simulink model "RoomRadiator_Compare"  (R2013b)
settings: Solver=ode23t  StartTime=0.0  StopTime=24*3600  RelTol=1e-3
undefined symbols (not defined in the file): density, heat_capacity
libraries: carnot x60, simulink x4, simulink_extras x2
settings Model: Creator=drhf  LastModifiedBy=drhf
settings OptimizationCC: ExpressionDepthLimit=2147483647
settings DebuggingCC: StateNameClashWarn=warning
settings GRTTargetCC: CombineOutputUpdateFcns=off  GRTInterface=on

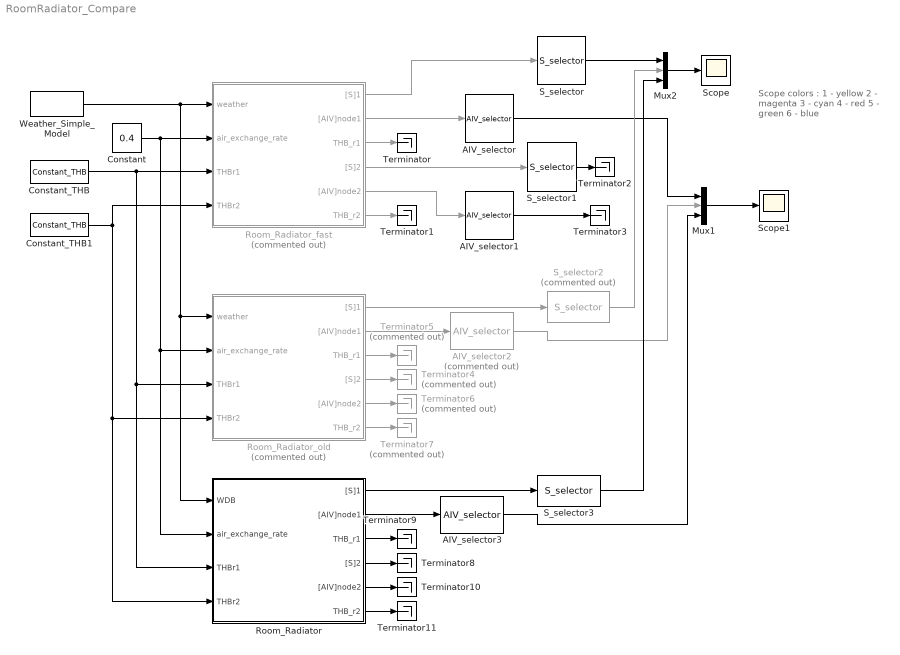
== system RoomRadiator_Compare ==
  note: Scope colors :
      | 1 - yellow
      | 2 - magenta
      | 3 - cyan
      | 4 - red
      | 5 - green
      | 6 - blue
  AIV_selector : carnot/Outputs/AIV_selector  e1=on  e2=on  e3=on  e4=off  e5=off  e6=off  e7=off  e8=off  e9=off
  AIV_selector1 : carnot/Outputs/AIV_selector  e1=on  e2=on  e3=on  e4=off  e5=off  e6=off  e7=off  e8=off  e9=off
  AIV_selector2 : carnot/Outputs/AIV_selector  Commented=on  e1=on  e2=on  e3=on  e4=off  e5=off  e6=off  e7=off  e8=off  e9=off
  AIV_selector3 : carnot/Outputs/AIV_selector  e1=on  e2=on  e3=on  e4=off  e5=off  e6=off  e7=off  e8=off  e9=off
  Constant : Constant  Value=0.4
  Constant_THB : carnot/Source/Simple/Constant_THB  t=30  mdot=600/3600  p=1e5  mID=No Pressure Drop  fluid=Water  mix=0  dia=0.02  hgt=0
  Constant_THB1 : carnot/Source/Simple/Constant_THB  t=40  mdot=600/3600  p=1e5  mID=No Pressure Drop  fluid=Water  mix=0  dia=0.02  hgt=0
  Mux1 : Mux  Inputs=3
  Mux2 : Mux  Inputs=3
  Room_Radiator : Subsystem  AncestorBlock=carnot/Load/Houses/Room_Radiator  mask(room){t0=20, temp_neighbour=20}
      mask prompts: t0 "start temperature of rooms in °C"; temp_neighbour "temperature of rooms above and below in °C"
      mask help:
      | The block models of a heat transfer characteristic of two neighbour rooms.
      | Use "look under mask" to set up the models parameters (initial conditions,
      | floors and wall characteristics...)
      mask init:
      | AIV_neighbour = [0 temp_neighbour temp_neighbour 0 0 0 0 0 0];
      | zonefloordist2grnd = 0;
      mask Help: web(fullfile(path_carnot('help'),'Room_Radiator.html'),'-helpbrowser')
      mask Display: plot(0,0,100,100,[30,30,60,60,30],[20,50,50,20,20],[47,47,56,56,47],[40,30,30,40,40],[42,42,34,34],[20,40,40,20],[62,45,28],[48,70,48])
  Room_Radiator_fast : Subsystem  Commented=on  AncestorBlock=carnot/Load/Houses/Room_Radiator  mask(room){t0=20, temp_neighbour=20}
      mask prompts: t0 "start temperature of rooms in °C"; temp_neighbour "temperature of rooms above and below in °C"
      mask help:
      | The block models of a heat transfer characteristic of two neighbour rooms.
      | Use "look under mask" to set up the models parameters (initial conditions,
      | floors and wall characteristics...)
      mask init:
      | AIV_neighbour = [0 temp_neighbour temp_neighbour 0 0 0 0 0 0];
      | zonefloordist2grnd = 0;
      mask Help: eval('man(''room_radiator'')')
      mask Display: plot(0,0,100,100,[30,30,60,60,30],[20,50,50,20,20],[47,47,56,56,47],[40,30,30,40,40],[42,42,34,34],[20,40,40,20],[62,45,28],[48,70,48])
  Room_Radiator_old : Subsystem  Commented=on  AncestorBlock=carnot/Load/Houses/Room_Radiator  mask(room){t0=20, temp_neighbour=20}
      mask prompts: t0 "start temperature of rooms in °C"; temp_neighbour "temperature of rooms above and below in °C"
      mask help:
      | The block models of a heat transfer characteristic of two neighbour rooms.
      | Use "look under mask" to set up the models parameters (initial conditions,
      | floors and wall characteristics...)
      mask init:
      | AIV_neighbour = [0 temp_neighbour temp_neighbour 0 0 0 0 0 0];
      | zonefloordist2grnd = 0;
      mask Help: eval('man(''room_radiator'')')
      mask Display: plot(0,0,100,100,[30,30,60,60,30],[20,50,50,20,20],[47,47,56,56,47],[40,30,30,40,40],[42,42,34,34],[20,40,40,20],[62,45,28],[48,70,48])
  S_selector : carnot/Outputs/S_selector  e1=off  e2=off  e3=off  e4=off  e5=off  e6=off  e7=on  e8=on  e9=off  e10=off  e11=off  e12=off  e13=off
  S_selector1 : carnot/Outputs/S_selector  e1=off  e2=off  e3=off  e4=off  e5=off  e6=off  e7=on  e8=on  e9=off  e10=off  e11=off  e12=off  e13=off
  S_selector2 : carnot/Outputs/S_selector  Commented=on  e1=off  e2=off  e3=off  e4=off  e5=off  e6=off  e7=on  e8=on  e9=off  e10=off  e11=off  e12=off  e13=off
  S_selector3 : carnot/Outputs/S_selector  e1=off  e2=off  e3=off  e4=off  e5=off  e6=off  e7=on  e8=on  e9=off  e10=off  e11=off  e12=off  e13=off
  Scope : Scope
      settings: YMin=0  YMax=12
  Scope1 : Scope
  Terminator{,1..3,8..11} (8 alike) : Terminator
  Terminator{4..7} (4 alike) : Terminator  Commented=on
  Weather_Simple_Model : carnot/Weather/Weather_Simple_Model  lat=60  Ibn=900  Idg=100  tamb=5  deltaTsky=-6  rh=50  precip="10e-3/24/3600           % 10 mm in 24 h"  cloud=0.125  p=1013e2  vw=1  wdir=270
  wires:
  Weather_Simple_Model/1 -> Room_Radiator_old/1(weather), Room_Radiator/1(WDB), Room_Radiator_fast/1(weather)
  Constant/1 -> Room_Radiator_old/2(air_exchange_rate), Room_Radiator/2(air_exchange_rate), Room_Radiator_fast/2(air_exchange_rate)
  Constant_THB/1 -> Room_Radiator_old/3(THBr1), Room_Radiator/3(THBr1), Room_Radiator_fast/3(THBr1)
  Constant_THB1/1 -> Room_Radiator_old/4(THBr2), Room_Radiator/4(THBr2), Room_Radiator_fast/4(THBr2)
  Room_Radiator_fast/1("[S]1") -> S_selector/1
  Room_Radiator_fast/2("[AIV]node1") -> AIV_selector/1
  Room_Radiator_fast/5("[AIV]node2") -> AIV_selector1/1
  Room_Radiator_fast/4("[S]2") -> S_selector1/1
  Room_Radiator_fast/3(THB_r1) -> Terminator/1
  Room_Radiator_fast/6(THB_r2) -> Terminator1/1
  Mux1/1 -> Scope1/1
  AIV_selector/1 -> Mux1/1
  S_selector1/1 -> Terminator2/1
  S_selector/1 -> Mux2/1
  Mux2/1 -> Scope/1
  Room_Radiator_old/1("[S]1") -> S_selector2/1
  S_selector2/1 -> Mux2/2
  AIV_selector1/1 -> Terminator3/1
  Room_Radiator_old/4("[S]2") -> Terminator4/1
  Room_Radiator_old/3(THB_r1) -> Terminator5/1
  Room_Radiator_old/5("[AIV]node2") -> Terminator6/1
  Room_Radiator_old/6(THB_r2) -> Terminator7/1
  Room_Radiator_old/2("[AIV]node1") -> AIV_selector2/1
  AIV_selector2/1 -> Mux1/2
  Room_Radiator/4("[S]2") -> Terminator8/1
  Room_Radiator/3(THB_r1) -> Terminator9/1
  Room_Radiator/5("[AIV]node2") -> Terminator10/1
  Room_Radiator/6(THB_r2) -> Terminator11/1
  Room_Radiator/2("[AIV]node1") -> AIV_selector3/1
  Room_Radiator/1("[S]1") -> S_selector3/1
  S_selector3/1 -> Mux2/3
  AIV_selector3/1 -> Mux1/3

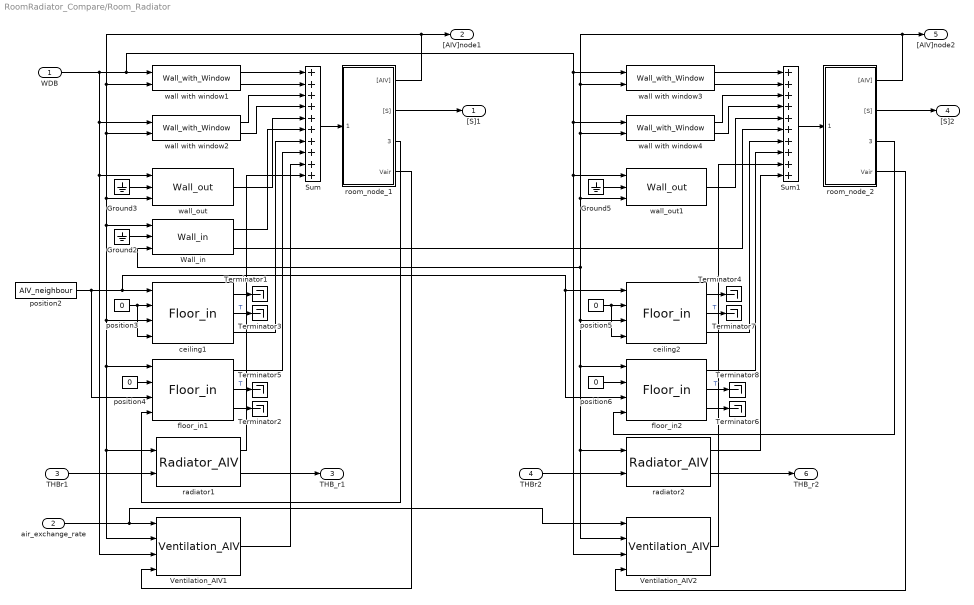
== system RoomRadiator_Compare/Room_Radiator ==
  WDB : Inport
  air_exchange_rate : Inport  Port=2
  THBr1 : Inport  Port=3
  THBr2 : Inport  Port=4
  Ground2 : Ground
  Ground3 : Ground
  Ground5 : Ground
  Sum : Sum  Inputs=10  SaturateOnIntegerOverflow=on  InputSameDT=on  OutDataTypeStr=Inherit: Same as first input
  Sum1 : Sum  Inputs=10  SaturateOnIntegerOverflow=on  InputSameDT=on  OutDataTypeStr=Inherit: Same as first input
  Terminator{1..8} (8 alike) : Terminator
  Ventilation_AIV1 : carnot/Source/Ventilation/Ventilation_AIV  co2=400
  Ventilation_AIV2 : carnot/Source/Ventilation/Ventilation_AIV  co2=400
  Wall_in : carnot/Load/Houses/wall_floor/Wall_in  wallsize=[2.5 5]  d=[0.015 0.38 0.02]  cond=[1.4 0.79 0.7]  cwall=[0.28 0.28 0.28]*3600  rho=[2000 1800 1400]  emission_in=0.96  dactive=-1  t0=20  tau=1000*3600
  ceiling1 : carnot/Load/Houses/wall_floor/Floor_in  wallsize=[5 5]  t0=20  d=[0.015 0.38 0.02]  cond=[1.4 0.79 0.7]  cwall=[0.28 0.28 0.28]*3600  rho=[2000 1800 1400]  misc=[.65 .65]  dactive=-1  tau=1000*3600
  ceiling2 : carnot/Load/Houses/wall_floor/Floor_in  wallsize=[5 5]  t0=20  d=[0.015 0.38 0.02]  cond=[1.4 0.79 0.7]  cwall=[0.28 0.28 0.28]*3600  rho=[2000 1800 1400]  misc=[.65 .65]  dactive=-1  tau=1000*3600
  floor_in1 : carnot/Load/Houses/wall_floor/Floor_in  wallsize=[5 5]  t0=20  d=[0.015 0.38 0.02]  cond=[1.4 0.79 0.7]  cwall=[0.28 0.28 0.28]*3600  rho=[2000 1800 1400]  misc=[.65 .65]  dactive=-1  tau=1000*3600
  floor_in2 : carnot/Load/Houses/wall_floor/Floor_in  wallsize=[5 5]  t0=20  d=[0.015 0.38 0.02]  cond=[1.4 0.79 0.7]  cwall=[0.28 0.28 0.28]*3600  rho=[2000 1800 1400]  misc=[.65 .65]  dactive=-1  tau=1000*3600
  position2 : Constant  Value=AIV_neighbour
  position{3..6} (4 alike) : Constant  Value=0
  radiator1 : carnot/Source/Heat_Exchanger/Radiator_AIV  pnom=500  dtnom=40  expo=1.3  mcap=5*4182  ra=0.47  tini=20  lin=0  qua=1000
  radiator2 : carnot/Source/Heat_Exchanger/Radiator_AIV  pnom=500  dtnom=40  expo=1.3  mcap=5*4182  ra=0.47  tini=20  lin=0  qua=1000
  room_node_1 : Subsystem  AncestorBlock=carnot/Load/Houses/room_node/Room_Node  mask(NODE){zoneairvolume=5*5*2.5, zoneheight=2.5, zonestartTEMP=20, zonestartWATER=55, timeconst=100, heatperfect=natural, lookuptime=[0 24]*3600, lookupvalue=[20 20], AirPressure=101300}
      mask prompts: zoneairvolume "SIZE: netto air volume >0, m^3"; zoneheight "SIZE: height of zone (floor - ceiling) >0, m"; zonestartTEMP "START TEMPERATURE: convective and radiative node, °C"; zonestartWATER "START AIR HUMIDITY: relative air humidity [0,100], %"; timeconst "timeconstant of radiative and convective node in s"; heatperfect "air temperature"; lookuptime "time vector for ideal profile [s]"; lookupvalue "values for ideal profile [degree centigrade]"; AirPressure "Air pressure for material properties in Pa"
      mask help:
      | This block delivers the energy consumption, temperature and air quality of a zone.
      | It is assumed that this node represents the center of a zone all connected sink and source blocks communicate with. Sink and source blocks are walls, windows, persons, heater etc..
      | Properties of air are calculated once at initialization (with node start temperature, humidity and air pressure).
      | [S] : input vector from sink blocks and source blocks
      | [AIV] : output vector with node temperature and air quality data.
      mask init:
      | CO2norm = 400*1e-6;
      | zoneairvolume = max(0.01, zoneairvolume);
      | zoneheight = max(0.01, zoneheight);
      | zonestartWATER = min(100, max(0, zonestartWATER));
      | zonestartWATER = rel_hum2x(zonestartTEMP, 10^5, zonestartWATER)*1.18*zoneairvolume; % kg H2O in zone volume (at 20°C)
      | zonestartCO2 = CO2norm*1.529*zoneairvolume; % kg CO2 in zone volume
      | zonestartAIR = 10^5*zoneairvolume/(287*(zonestartTEMP+273)); % kg AIR in zone volume
      mask Help: web(fullfile(path_carnot('help'),'Room_Node.html'),'-helpbrowser')
      mask TypeOptions heatperfect: natural | ideal profile (for heating demand)
  room_node_2 : Subsystem  AncestorBlock=carnot/Load/Houses/room_node/Room_Node  mask(NODE){zoneairvolume=5*5*2.5, zoneheight=2.5, zonestartTEMP=20, zonestartWATER=55, timeconst=100, heatperfect=natural, lookuptime=[0 24]*3600, lookupvalue=[20 20], AirPressure=101300}
      mask prompts: zoneairvolume "SIZE: netto air volume >0, m^3"; zoneheight "SIZE: height of zone (floor - ceiling) >0, m"; zonestartTEMP "START TEMPERATURE: convective and radiative node, °C"; zonestartWATER "START AIR HUMIDITY: relative air humidity [0,100], %"; timeconst "timeconstant of radiative and convective node in s"; heatperfect "air temperature"; lookuptime "time vector for ideal profile [s]"; lookupvalue "values for ideal profile [degree centigrade]"; AirPressure "Air pressure for material properties in Pa"
      mask help:
      | This block delivers the energy consumption, temperature and air quality of a zone.
      | It is assumed that this node represents the center of a zone all connected sink and source blocks communicate with. Sink and source blocks are walls, windows, persons, heater etc..
      | Properties of air are calculated once at initialization (with node start temperature, humidity and air pressure).
      | [S] : input vector from sink blocks and source blocks
      | [AIV] : output vector with node temperature and air quality data.
      mask init: same as RoomRadiator_Compare/Room_Radiator/room_node_1
      mask Help: web(fullfile(path_carnot('help'),'Room_Node.html'),'-helpbrowser')
      mask TypeOptions heatperfect: natural | ideal profile (for heating demand)
  wall with window1 : carnot/Load/Houses/wall_floor/Wall_with_Window  wallsize=[2.5 5]  windowsize=[1 2]  frame=0.1  pos=90  t0=20  tau=1000*3600  g=0.7
  wall with window2 : carnot/Load/Houses/wall_floor/Wall_with_Window  wallsize=[2.5 5]  windowsize=[1 2]  frame=0.1  pos=0  t0=20  tau=1000*3600  g=0.7
  wall with window3 : carnot/Load/Houses/wall_floor/Wall_with_Window  wallsize=[2.5 5]  windowsize=[1 2]  frame=0.1  pos=-90  t0=20  tau=1000*3600  g=0.7
  wall with window4 : carnot/Load/Houses/wall_floor/Wall_with_Window  wallsize=[2.5 5]  windowsize=[1 2]  frame=0.1  pos=0  t0=20  tau=1000*3600  g=0.7
  wall_out : carnot/Load/Houses/wall_floor/Wall_out  wallsize=[2.5 5]  pos=180  t0=20  d=[0.1 0.38]  cond=[0.04 0.79]  cwall=[0.28 0.28]*3600  rho=[900 1800]  reflectground=0.2  abs_emiss=[0.65 0.97 0.96]  tau=1000*3600  dactive=-1
  wall_out1 : carnot/Load/Houses/wall_floor/Wall_out  wallsize=[2.5 5]  pos=180  t0=20  d=[0.1 0.38]  cond=[0.04 0.79]  cwall=[0.28 0.28]*3600  rho=[900 1800]  reflectground=0.2  abs_emiss=[0.65 0.97 0.96]  tau=1000*3600  dactive=-1
  "[S]1" : Outport
  "[AIV]node1" : Outport  Port=2
  THB_r1 : Outport  Port=3
  "[S]2" : Outport  Port=4
  "[AIV]node2" : Outport  Port=5
  THB_r2 : Outport  Port=6
  wires:
  Sum1/1 -> room_node_2/1(sum([S]))
  Sum/1 -> room_node_1/1(sum([S]))
  radiator2/1 -> Sum1/10
  radiator1/1 -> Sum/10
  position6/1 -> floor_in2/2
  position4/1 -> floor_in1/2
  floor_in1/2 -> Terminator5/1  "T"
  floor_in2/2 -> Terminator8/1  "T"
  room_node_2/1("[AIV]") -> "[AIV]node2"/1, wall with window3/2, wall with window4/2, Wall_in/3, ceiling2/3, Ventilation_AIV2/2, radiator2/1, floor_in2/1, wall_out1/3
  room_node_1/1("[AIV]") -> "[AIV]node1"/1, wall_out/3, Wall_in/1, Ventilation_AIV1/2, radiator1/1, floor_in1/1, ceiling1/3, wall with window2/2, wall with window1/2
  air_exchange_rate/1 -> Ventilation_AIV2/1, Ventilation_AIV1/1
  Wall_in/2 -> Sum1/6
  Ground5/1 -> wall_out1/2
  room_node_2/3(Qdot_sol) -> floor_in2/4
  room_node_2/4(Vair) -> Ventilation_AIV2/4
  radiator2/2 -> THB_r2/1
  THBr2/1 -> radiator2/2
  Ventilation_AIV2/1 -> Sum1/9
  ceiling2/3 -> Sum1/7
  floor_in2/1 -> Sum1/8
  position5/1 -> ceiling2/2, ceiling2/4
  floor_in2/3 -> Terminator6/1
  ceiling2/2 -> Terminator7/1  "T"
  ceiling2/1 -> Terminator4/1
  room_node_2/2("[S]") -> "[S]2"/1
  wall with window4/2 -> Sum1/4
  wall_out1/1 -> Sum1/5
  wall with window4/1 -> Sum1/3
  wall with window3/2 -> Sum1/2
  wall with window3/1 -> Sum1/1
  position2/1 -> floor_in2/3, ceiling2/1, ceiling1/1, floor_in1/3
  Ground3/1 -> wall_out/2
  Ground2/1 -> Wall_in/2
  room_node_1/3(Qdot_sol) -> floor_in1/4
  room_node_1/4(Vair) -> Ventilation_AIV1/4
  radiator1/2 -> THB_r1/1
  THBr1/1 -> radiator1/2
  Ventilation_AIV1/1 -> Sum/9
  ceiling1/3 -> Sum/7
  floor_in1/1 -> Sum/8
  position3/1 -> ceiling1/4, ceiling1/2
  floor_in1/3 -> Terminator2/1
  ceiling1/2 -> Terminator3/1  "T"
  ceiling1/1 -> Terminator1/1
  room_node_1/2("[S]") -> "[S]1"/1
  wall with window2/2 -> Sum/4
  wall_out/1 -> Sum/5
  wall with window2/1 -> Sum/3
  wall with window1/2 -> Sum/2
  wall with window1/1 -> Sum/1
  WDB/1 -> wall with window3/1, wall with window4/1, Ventilation_AIV2/3, wall_out1/1, wall with window1/1, Ventilation_AIV1/3, wall_out/1, wall with window2/1
  Wall_in/1 -> Sum/6

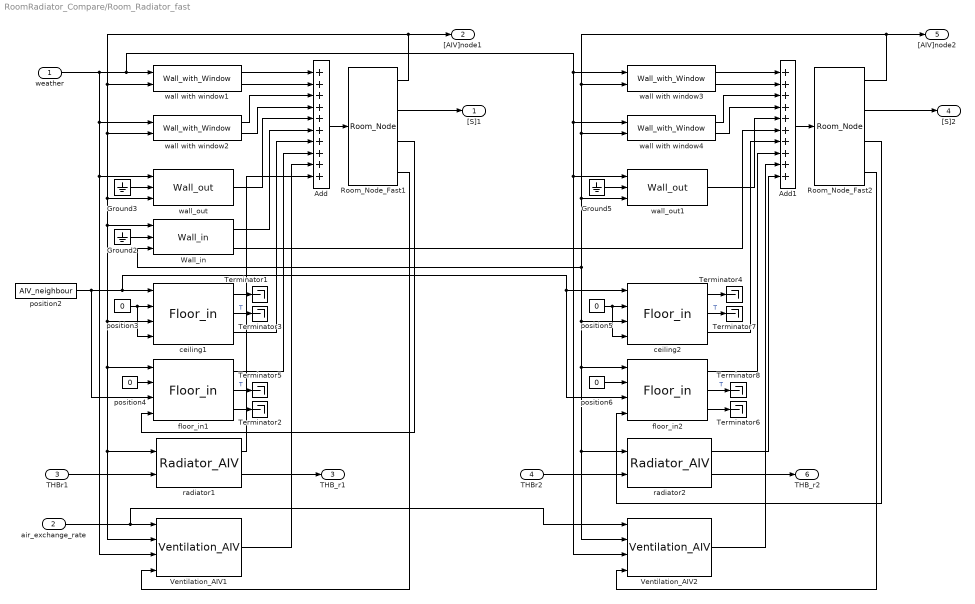
== system RoomRadiator_Compare/Room_Radiator_fast ==
  weather : Inport
  air_exchange_rate : Inport  Port=2
  THBr1 : Inport  Port=3
  THBr2 : Inport  Port=4
  Add : Sum  Inputs=10
  Add1 : Sum  Inputs=10
  Ground2 : Ground
  Ground3 : Ground
  Ground5 : Ground
  Room_Node_Fast1 : carnot/Load/Houses/room_node/Room_Node  zoneairvolume=5*5*2.5  zoneheight=2.5  zonestartTEMP=20  zonestartWATER=55  timeconst=100  heatperfect=natural  lookuptime=[0 7 7 20 20 24]*3600  lookupvalue=[18 18 20 20 18 18]  AirPressure=101300
  Room_Node_Fast2 : carnot/Load/Houses/room_node/Room_Node  zoneairvolume=5*5*2.5  zoneheight=2.5  zonestartTEMP=20  zonestartWATER=55  timeconst=100  heatperfect=natural  lookuptime=[0 7 7 20 20 24]*3600  lookupvalue=[18 18 20 20 18 18]  AirPressure=101300
  Terminator{1..8} (8 alike) : Terminator
  Ventilation_AIV1 : carnot/Source/Ventilation/Ventilation_AIV  co2=400
  Ventilation_AIV2 : carnot/Source/Ventilation/Ventilation_AIV  co2=400
  Wall_in : carnot/Load/Houses/wall_floor/Wall_in  wallsize=[2.5 5]  d=[0.015 0.38 0.02]  cond=[1.4 0.79 0.7]  cwall=[0.28 0.28 0.28]*3600  rho=[2000 1800 1400]  emission_in=0.96  dactive=-1  t0=20  tau=1000*3600
  ceiling1 : carnot/Load/Houses/wall_floor/Floor_in  wallsize=[5 5]  t0=20  d=[0.015 0.38 0.02]  cond=[1.4 0.79 0.7]  cwall=[0.28 0.28 0.28]*3600  rho=[2000 1800 1400]  misc=[.65 .65]  dactive=-1  tau=1000*3600
  ceiling2 : carnot/Load/Houses/wall_floor/Floor_in  wallsize=[5 5]  t0=20  d=[0.015 0.38 0.02]  cond=[1.4 0.79 0.7]  cwall=[0.28 0.28 0.28]*3600  rho=[2000 1800 1400]  misc=[.65 .65]  dactive=-1  tau=1000*3600
  floor_in1 : carnot/Load/Houses/wall_floor/Floor_in  wallsize=[5 5]  t0=20  d=[0.015 0.38 0.02]  cond=[1.4 0.79 0.7]  cwall=[0.28 0.28 0.28]*3600  rho=[2000 1800 1400]  misc=[.65 .65]  dactive=-1  tau=1000*3600
  floor_in2 : carnot/Load/Houses/wall_floor/Floor_in  wallsize=[5 5]  t0=20  d=[0.015 0.38 0.02]  cond=[1.4 0.79 0.7]  cwall=[0.28 0.28 0.28]*3600  rho=[2000 1800 1400]  misc=[.65 .65]  dactive=-1  tau=1000*3600
  position2 : Constant  Value=AIV_neighbour
  position{3..6} (4 alike) : Constant  Value=0
  radiator1 : carnot/Source/Heat_Exchanger/Radiator_AIV  pnom=500  dtnom=40  expo=1.3  mcap=5*4182  ra=0.47  tini=20  lin=0  qua=1000
  radiator2 : carnot/Source/Heat_Exchanger/Radiator_AIV  pnom=500  dtnom=40  expo=1.3  mcap=5*4182  ra=0.47  tini=20  lin=0  qua=1000
  wall with window1 : carnot/Load/Houses/wall_floor/Wall_with_Window  wallsize=[2.5 5]  windowsize=[1 2]  frame=0.1  pos=90  t0=20  tau=1000*3600  g=0.7
  wall with window2 : carnot/Load/Houses/wall_floor/Wall_with_Window  wallsize=[2.5 5]  windowsize=[1 2]  frame=0.1  pos=0  t0=20  tau=1000*3600  g=0.7
  wall with window3 : carnot/Load/Houses/wall_floor/Wall_with_Window  wallsize=[2.5 5]  windowsize=[1 2]  frame=0.1  pos=-90  t0=20  tau=1000*3600  g=0.7
  wall with window4 : carnot/Load/Houses/wall_floor/Wall_with_Window  wallsize=[2.5 5]  windowsize=[1 2]  frame=0.1  pos=0  t0=20  tau=1000*3600  g=0.7
  wall_out : carnot/Load/Houses/wall_floor/Wall_out  wallsize=[2.5 5]  pos=180  t0=20  d=[0.1 0.38]  cond=[0.04 0.79]  cwall=[0.28 0.28]*3600  rho=[900 1800]  reflectground=0.2  abs_emiss=[0.65 0.97 0.96]  tau=1000*3600  dactive=-1
  wall_out1 : carnot/Load/Houses/wall_floor/Wall_out  wallsize=[2.5 5]  pos=180  t0=20  d=[0.1 0.38]  cond=[0.04 0.79]  cwall=[0.28 0.28]*3600  rho=[900 1800]  reflectground=0.2  abs_emiss=[0.65 0.97 0.96]  tau=1000*3600  dactive=-1
  "[S]1" : Outport
  "[AIV]node1" : Outport  Port=2
  THB_r1 : Outport  Port=3
  "[S]2" : Outport  Port=4
  "[AIV]node2" : Outport  Port=5
  THB_r2 : Outport  Port=6
  wires:
  radiator2/1 -> Add1/10
  radiator1/1 -> Add/10
  position6/1 -> floor_in2/2
  position4/1 -> floor_in1/2
  floor_in1/2 -> Terminator5/1  "T"
  floor_in2/2 -> Terminator8/1  "T"
  Room_Node_Fast2/1 -> wall with window3/2, wall with window4/2, Wall_in/3, ceiling2/3, Ventilation_AIV2/2, radiator2/1, floor_in2/1, wall_out1/3, "[AIV]node2"/1
  Room_Node_Fast1/1 -> wall_out/3, Wall_in/1, Ventilation_AIV1/2, radiator1/1, floor_in1/1, ceiling1/3, wall with window2/2, wall with window1/2, "[AIV]node1"/1
  air_exchange_rate/1 -> Ventilation_AIV2/1, Ventilation_AIV1/1
  Wall_in/2 -> Add1/6
  Ground5/1 -> wall_out1/2
  Room_Node_Fast2/3 -> floor_in2/4
  Room_Node_Fast2/4 -> Ventilation_AIV2/4
  radiator2/2 -> THB_r2/1
  THBr2/1 -> radiator2/2
  Ventilation_AIV2/1 -> Add1/9
  ceiling2/3 -> Add1/7
  floor_in2/1 -> Add1/8
  position5/1 -> ceiling2/2, ceiling2/4
  floor_in2/3 -> Terminator6/1
  ceiling2/2 -> Terminator7/1  "T"
  ceiling2/1 -> Terminator4/1
  Room_Node_Fast2/2 -> "[S]2"/1
  wall with window4/2 -> Add1/4
  wall_out1/1 -> Add1/5
  wall with window4/1 -> Add1/3
  wall with window3/2 -> Add1/2
  wall with window3/1 -> Add1/1
  position2/1 -> floor_in2/3, ceiling2/1, ceiling1/1, floor_in1/3
  Ground3/1 -> wall_out/2
  Ground2/1 -> Wall_in/2
  Room_Node_Fast1/3 -> floor_in1/4
  Room_Node_Fast1/4 -> Ventilation_AIV1/4
  radiator1/2 -> THB_r1/1
  THBr1/1 -> radiator1/2
  Ventilation_AIV1/1 -> Add/9
  ceiling1/3 -> Add/7
  floor_in1/1 -> Add/8
  position3/1 -> ceiling1/4, ceiling1/2
  floor_in1/3 -> Terminator2/1
  ceiling1/2 -> Terminator3/1  "T"
  ceiling1/1 -> Terminator1/1
  Room_Node_Fast1/2 -> "[S]1"/1
  wall with window2/2 -> Add/4
  wall_out/1 -> Add/5
  wall with window2/1 -> Add/3
  wall with window1/2 -> Add/2
  wall with window1/1 -> Add/1
  weather/1 -> wall with window3/1, wall with window4/1, Ventilation_AIV2/3, wall_out1/1, wall with window1/1, Ventilation_AIV1/3, wall_out/1, wall with window2/1
  Wall_in/1 -> Add/6
  Add/1 -> Room_Node_Fast1/1
  Add1/1 -> Room_Node_Fast2/1

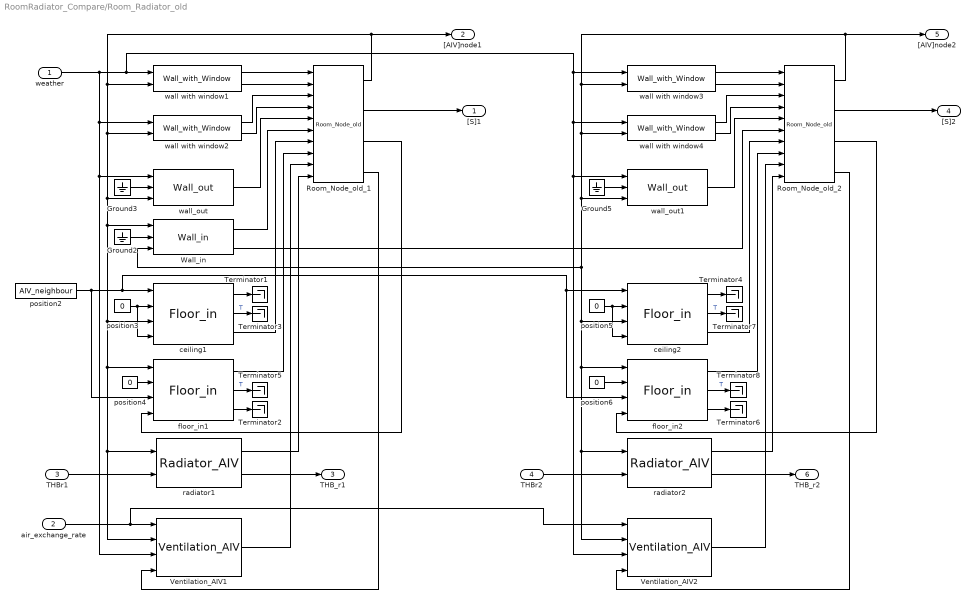
== system RoomRadiator_Compare/Room_Radiator_old ==
  weather : Inport
  air_exchange_rate : Inport  Port=2
  THBr1 : Inport  Port=3
  THBr2 : Inport  Port=4
  Ground2 : Ground
  Ground3 : Ground
  Ground5 : Ground
  Room_Node_old_1 : carnot/Load/Houses/room_node/Room_Node_old  SystemSampleTime=-1  zoneairvolume=5*5*2.5  zoneheight=2.5  zonestartTEMP=20  zonestartWATER=55  timeconst=100  heatperfect=natural  lookuptime=[0 7 7 20 20 24]*3600  lookupvalue=[18 18 20 20 18 18]
  Room_Node_old_2 : carnot/Load/Houses/room_node/Room_Node_old  SystemSampleTime=-1  zoneairvolume=5*5*2.5  zoneheight=2.5  zonestartTEMP=20  zonestartWATER=55  timeconst=100  heatperfect=natural  lookuptime=[0 7 7 20 20 24]*3600  lookupvalue=[18 18 20 20 18 18]
  Terminator{1..8} (8 alike) : Terminator
  Ventilation_AIV1 : carnot/Source/Ventilation/Ventilation_AIV  co2=400
  Ventilation_AIV2 : carnot/Source/Ventilation/Ventilation_AIV  co2=400
  Wall_in : carnot/Load/Houses/wall_floor/Wall_in  wallsize=[2.5 5]  d=[0.015 0.38 0.02]  cond=[1.4 0.79 0.7]  cwall=[0.28 0.28 0.28]*3600  rho=[2000 1800 1400]  emission_in=0.96  dactive=-1  t0=20  tau=1000*3600
  ceiling1 : carnot/Load/Houses/wall_floor/Floor_in  wallsize=[5 5]  t0=20  d=[0.015 0.38 0.02]  cond=[1.4 0.79 0.7]  cwall=[0.28 0.28 0.28]*3600  rho=[2000 1800 1400]  misc=[.65 .65]  dactive=-1  tau=1000*3600
  ceiling2 : carnot/Load/Houses/wall_floor/Floor_in  wallsize=[5 5]  t0=20  d=[0.015 0.38 0.02]  cond=[1.4 0.79 0.7]  cwall=[0.28 0.28 0.28]*3600  rho=[2000 1800 1400]  misc=[.65 .65]  dactive=-1  tau=1000*3600
  floor_in1 : carnot/Load/Houses/wall_floor/Floor_in  wallsize=[5 5]  t0=20  d=[0.015 0.38 0.02]  cond=[1.4 0.79 0.7]  cwall=[0.28 0.28 0.28]*3600  rho=[2000 1800 1400]  misc=[.65 .65]  dactive=-1  tau=1000*3600
  floor_in2 : carnot/Load/Houses/wall_floor/Floor_in  wallsize=[5 5]  t0=20  d=[0.015 0.38 0.02]  cond=[1.4 0.79 0.7]  cwall=[0.28 0.28 0.28]*3600  rho=[2000 1800 1400]  misc=[.65 .65]  dactive=-1  tau=1000*3600
  position2 : Constant  Value=AIV_neighbour
  position{3..6} (4 alike) : Constant  Value=0
  radiator1 : carnot/Source/Heat_Exchanger/Radiator_AIV  pnom=500  dtnom=40  expo=1.3  mcap=5*4182  ra=0.47  tini=20  lin=0  qua=1000
  radiator2 : carnot/Source/Heat_Exchanger/Radiator_AIV  pnom=500  dtnom=40  expo=1.3  mcap=5*4182  ra=0.47  tini=20  lin=0  qua=1000
  wall with window1 : carnot/Load/Houses/wall_floor/Wall_with_Window  wallsize=[2.5 5]  windowsize=[1 2]  frame=0.1  pos=90  t0=20  tau=1000*3600  g=0.7
  wall with window2 : carnot/Load/Houses/wall_floor/Wall_with_Window  wallsize=[2.5 5]  windowsize=[1 2]  frame=0.1  pos=0  t0=20  tau=1000*3600  g=0.7
  wall with window3 : carnot/Load/Houses/wall_floor/Wall_with_Window  wallsize=[2.5 5]  windowsize=[1 2]  frame=0.1  pos=-90  t0=20  tau=1000*3600  g=0.7
  wall with window4 : carnot/Load/Houses/wall_floor/Wall_with_Window  wallsize=[2.5 5]  windowsize=[1 2]  frame=0.1  pos=0  t0=20  tau=1000*3600  g=0.7
  wall_out : carnot/Load/Houses/wall_floor/Wall_out  wallsize=[2.5 5]  pos=180  t0=20  d=[0.1 0.38]  cond=[0.04 0.79]  cwall=[0.28 0.28]*3600  rho=[900 1800]  reflectground=0.2  abs_emiss=[0.65 0.97 0.96]  tau=1000*3600  dactive=-1
  wall_out1 : carnot/Load/Houses/wall_floor/Wall_out  wallsize=[2.5 5]  pos=180  t0=20  d=[0.1 0.38]  cond=[0.04 0.79]  cwall=[0.28 0.28]*3600  rho=[900 1800]  reflectground=0.2  abs_emiss=[0.65 0.97 0.96]  tau=1000*3600  dactive=-1
  "[S]1" : Outport
  "[AIV]node1" : Outport  Port=2
  THB_r1 : Outport  Port=3
  "[S]2" : Outport  Port=4
  "[AIV]node2" : Outport  Port=5
  THB_r2 : Outport  Port=6
  wires:
  Wall_in/1 -> Room_Node_old_1/6
  weather/1 -> wall with window2/1, wall_out/1, Ventilation_AIV1/3, wall with window1/1, wall_out1/1, Ventilation_AIV2/3, wall with window4/1, wall with window3/1
  wall with window1/1 -> Room_Node_old_1/1
  wall with window1/2 -> Room_Node_old_1/2
  wall with window2/1 -> Room_Node_old_1/3
  wall_out/1 -> Room_Node_old_1/5
  wall with window2/2 -> Room_Node_old_1/4
  Room_Node_old_1/2 -> "[S]1"/1
  ceiling1/1 -> Terminator1/1
  ceiling1/2 -> Terminator3/1  "T"
  floor_in1/3 -> Terminator2/1
  position3/1 -> ceiling1/2, ceiling1/4
  floor_in1/1 -> Room_Node_old_1/8
  ceiling1/3 -> Room_Node_old_1/7
  Ventilation_AIV1/1 -> Room_Node_old_1/9
  THBr1/1 -> radiator1/2
  radiator1/2 -> THB_r1/1
  Room_Node_old_1/4 -> Ventilation_AIV1/4
  Room_Node_old_1/3 -> floor_in1/4
  Ground2/1 -> Wall_in/2
  Ground3/1 -> wall_out/2
  position2/1 -> floor_in1/3, ceiling1/1, ceiling2/1, floor_in2/3
  wall with window3/1 -> Room_Node_old_2/1
  wall with window3/2 -> Room_Node_old_2/2
  wall with window4/1 -> Room_Node_old_2/3
  wall_out1/1 -> Room_Node_old_2/5
  wall with window4/2 -> Room_Node_old_2/4
  Room_Node_old_2/2 -> "[S]2"/1
  ceiling2/1 -> Terminator4/1
  ceiling2/2 -> Terminator7/1  "T"
  floor_in2/3 -> Terminator6/1
  position5/1 -> ceiling2/4, ceiling2/2
  floor_in2/1 -> Room_Node_old_2/8
  ceiling2/3 -> Room_Node_old_2/7
  Ventilation_AIV2/1 -> Room_Node_old_2/9
  THBr2/1 -> radiator2/2
  radiator2/2 -> THB_r2/1
  Room_Node_old_2/4 -> Ventilation_AIV2/4
  Room_Node_old_2/3 -> floor_in2/4
  Ground5/1 -> wall_out1/2
  Wall_in/2 -> Room_Node_old_2/6
  air_exchange_rate/1 -> Ventilation_AIV1/1, Ventilation_AIV2/1
  Room_Node_old_1/1 -> wall with window1/2, wall with window2/2, ceiling1/3, floor_in1/1, radiator1/1, Ventilation_AIV1/2, Wall_in/1, wall_out/3, "[AIV]node1"/1
  Room_Node_old_2/1 -> wall_out1/3, floor_in2/1, radiator2/1, Ventilation_AIV2/2, ceiling2/3, Wall_in/3, wall with window4/2, wall with window3/2, "[AIV]node2"/1
  floor_in2/2 -> Terminator8/1  "T"
  floor_in1/2 -> Terminator5/1  "T"
  position4/1 -> floor_in1/2
  position6/1 -> floor_in2/2
  radiator1/1 -> Room_Node_old_1/10
  radiator2/1 -> Room_Node_old_2/10

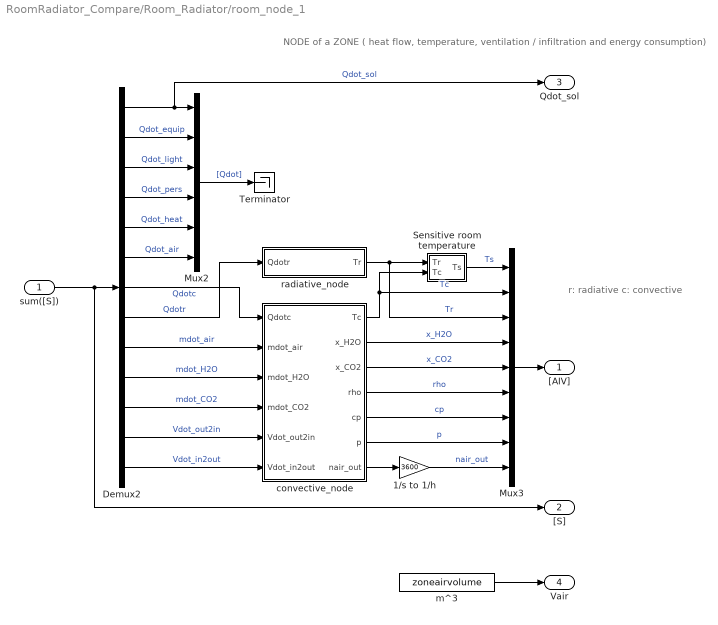
== system RoomRadiator_Compare/Room_Radiator/room_node_1 ==
  note: NODE of a ZONE ( heat flow, temperature, ventilation / infiltration and energy consumption)
  note: r: radiative
      | c: convective
  sum([S]) : Inport
  1/s to 1/h : Gain  Gain=3600  SaturateOnIntegerOverflow=on  OutDataTypeStr=Inherit: Same as input  ParamDataTypeStr=Inherit: Same as input
  Demux2 : Demux  Outputs=13
  Mux2 : Mux  Inputs=6
  Mux3 : Mux  Inputs=9
  Sensitive room temperature : Subsystem  mask(SENSITIVE TEMPERATURE){share_c=47}
      mask prompts: share_c "SHARE of convective sensitivity, [0,100%]:"
      mask help:
      | This block merges the convective and radiative zone node temperature to the SENSITIVE ZONE TEMPERATURE (weighted arithmetic average of both components).
      |
      | [T] = [Tc; Tr]:  temperature vector of node, °C
      | Ts:              sensitive zone temperature, °C
      mask init:
      | blockname = gcb;
      | 
      | if (length(share_c)~=1) error(['PARAMETERS block "' blockname ': "SHARE of ..." must have only 1 entry !']); end;
      | if (share_c<0) | (share_c>100) error(['PARAMETERS block "' blockname '" : "SHARE of ..." must be within [0, 100%] !']); end;
      | share_c = share_c/100;
  Terminator : Terminator
  convective_node : Subsystem
  m^3 : Constant  Value=zoneairvolume
  radiative_node : Subsystem
  "[AIV]" : Outport
  "[S]" : Outport  Port=2
  Qdot_sol : Outport  Port=3
  Vair : Outport  Port=4
  wires:
  Sensitive room temperature/1(Ts) -> Mux3/1  "Ts"
  Mux3/1 -> "[AIV]"/1
  Demux2/13 -> convective_node/6(Vdot_in2out)  "Vdot_in2out"
  Demux2/12 -> convective_node/5(Vdot_out2in)  "Vdot_out2in"
  Demux2/11 -> convective_node/4(mdot_CO2)  "mdot_CO2"
  Demux2/10 -> convective_node/3(mdot_H2O)  "mdot_H2O"
  Demux2/9 -> convective_node/2(mdot_air)  "mdot_air"
  radiative_node/1(Tr) -> Mux3/3, Sensitive room temperature/1(Tr)  "Tr"
  convective_node/1(Tc) -> Mux3/2, Sensitive room temperature/2(Tc)  "Tc"
  convective_node/7(nair_out) -> 1/s to 1/h/1
  convective_node/4(rho) -> Mux3/6  "rho"
  convective_node/5(cp) -> Mux3/7  "cp"
  convective_node/6(p) -> Mux3/8  "p"
  convective_node/3(x_CO2) -> Mux3/5  "x_CO2"
  convective_node/2(x_H2O) -> Mux3/4  "x_H2O"
  1/s to 1/h/1 -> Mux3/9  "nair_out"
  Demux2/1 -> Qdot_sol/1, Mux2/1  "Qdot_sol"
  Demux2/2 -> Mux2/2  "Qdot_equip"
  Demux2/3 -> Mux2/3  "Qdot_light"
  Demux2/4 -> Mux2/4  "Qdot_pers"
  Demux2/5 -> Mux2/5  "Qdot_heat"
  Demux2/6 -> Mux2/6  "Qdot_air"
  Demux2/7 -> convective_node/1(Qdotc)  "Qdotc"
  Demux2/8 -> radiative_node/1(Qdotr)  "Qdotr"
  sum([S])/1 -> Demux2/1, "[S]"/1
  Mux2/1 -> Terminator/1  "[Qdot]"
  m^3/1 -> Vair/1

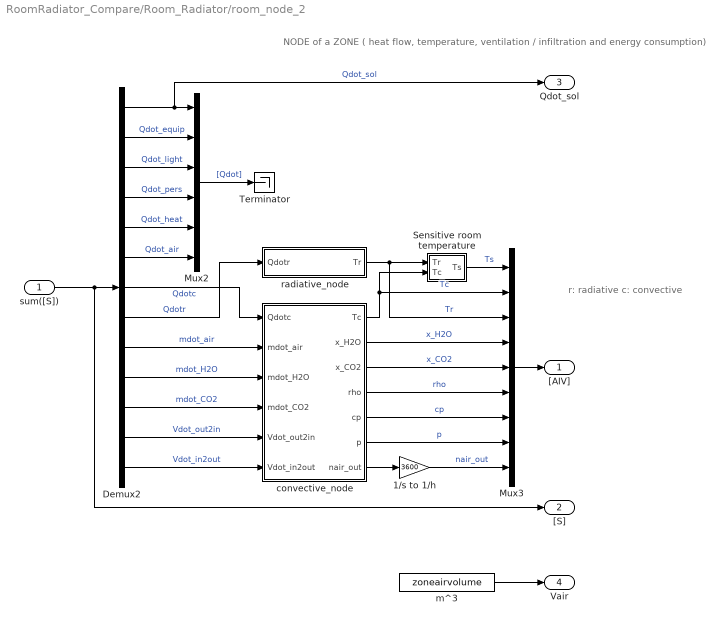
== system RoomRadiator_Compare/Room_Radiator/room_node_2 ==
  note: NODE of a ZONE ( heat flow, temperature, ventilation / infiltration and energy consumption)
  note: r: radiative
      | c: convective
  sum([S]) : Inport
  1/s to 1/h : Gain  Gain=3600  SaturateOnIntegerOverflow=on  OutDataTypeStr=Inherit: Same as input  ParamDataTypeStr=Inherit: Same as input
  Demux2 : Demux  Outputs=13
  Mux2 : Mux  Inputs=6
  Mux3 : Mux  Inputs=9
  Sensitive room temperature : Subsystem  mask(SENSITIVE TEMPERATURE){share_c=47}
      mask prompts: share_c "SHARE of convective sensitivity, [0,100%]:"
      mask help:
      | This block merges the convective and radiative zone node temperature to the SENSITIVE ZONE TEMPERATURE (weighted arithmetic average of both components).
      |
      | [T] = [Tc; Tr]:  temperature vector of node, °C
      | Ts:              sensitive zone temperature, °C
      mask init: same as RoomRadiator_Compare/Room_Radiator/room_node_1/Sensitive room temperature
  Terminator : Terminator
  convective_node : Subsystem
  m^3 : Constant  Value=zoneairvolume
  radiative_node : Subsystem
  "[AIV]" : Outport
  "[S]" : Outport  Port=2
  Qdot_sol : Outport  Port=3
  Vair : Outport  Port=4
  wires:
  Sensitive room temperature/1(Ts) -> Mux3/1  "Ts"
  Mux3/1 -> "[AIV]"/1
  Demux2/13 -> convective_node/6(Vdot_in2out)  "Vdot_in2out"
  Demux2/12 -> convective_node/5(Vdot_out2in)  "Vdot_out2in"
  Demux2/11 -> convective_node/4(mdot_CO2)  "mdot_CO2"
  Demux2/10 -> convective_node/3(mdot_H2O)  "mdot_H2O"
  Demux2/9 -> convective_node/2(mdot_air)  "mdot_air"
  radiative_node/1(Tr) -> Mux3/3, Sensitive room temperature/1(Tr)  "Tr"
  convective_node/1(Tc) -> Mux3/2, Sensitive room temperature/2(Tc)  "Tc"
  convective_node/7(nair_out) -> 1/s to 1/h/1
  convective_node/4(rho) -> Mux3/6  "rho"
  convective_node/5(cp) -> Mux3/7  "cp"
  convective_node/6(p) -> Mux3/8  "p"
  convective_node/3(x_CO2) -> Mux3/5  "x_CO2"
  convective_node/2(x_H2O) -> Mux3/4  "x_H2O"
  1/s to 1/h/1 -> Mux3/9  "nair_out"
  Demux2/1 -> Qdot_sol/1, Mux2/1  "Qdot_sol"
  Demux2/2 -> Mux2/2  "Qdot_equip"
  Demux2/3 -> Mux2/3  "Qdot_light"
  Demux2/4 -> Mux2/4  "Qdot_pers"
  Demux2/5 -> Mux2/5  "Qdot_heat"
  Demux2/6 -> Mux2/6  "Qdot_air"
  Demux2/7 -> convective_node/1(Qdotc)  "Qdotc"
  Demux2/8 -> radiative_node/1(Qdotr)  "Qdotr"
  sum([S])/1 -> Demux2/1, "[S]"/1
  Mux2/1 -> Terminator/1  "[Qdot]"
  m^3/1 -> Vair/1

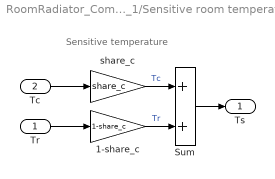
== system RoomRadiator_Compare/Room_Radiator/room_node_1/Sensitive room temperature ==
  note: Sensitive temperature
  Tr : Inport
  Tc : Inport  Port=2
  1-share_c : Gain  Gain=1-share_c  SaturateOnIntegerOverflow=on  OutDataTypeStr=Inherit: Same as input  ParamDataTypeStr=Inherit: Same as input
  Sum : Sum  SaturateOnIntegerOverflow=on  InputSameDT=on  OutDataTypeStr=Inherit: Same as first input
  share_c : Gain  Gain=share_c  SaturateOnIntegerOverflow=on  OutDataTypeStr=Inherit: Same as input  ParamDataTypeStr=Inherit: Same as input
  Ts : Outport
  wires:
  Tr/1 -> 1-share_c/1
  Tc/1 -> share_c/1
  share_c/1 -> Sum/1  "Tc"
  1-share_c/1 -> Sum/2  "Tr"
  Sum/1 -> Ts/1

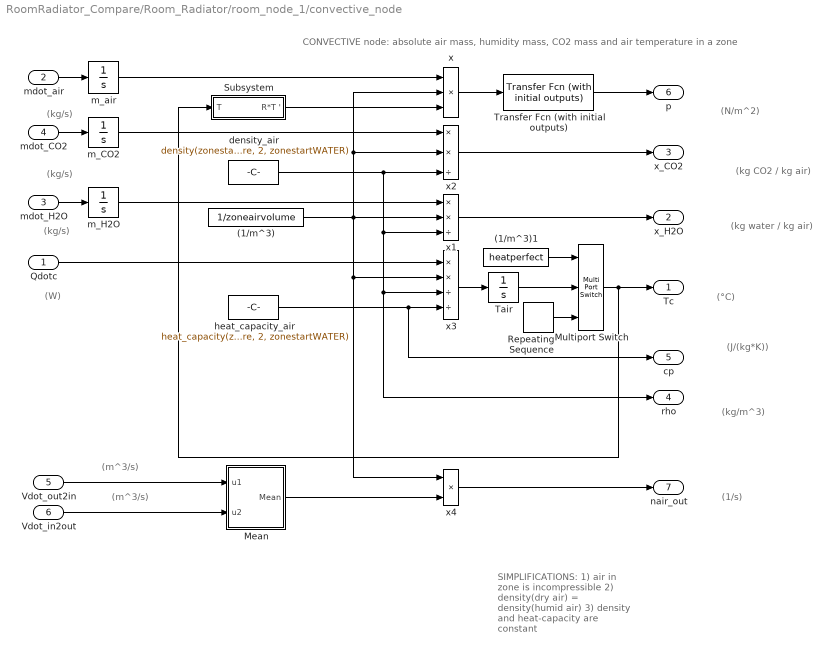
== system RoomRadiator_Compare/Room_Radiator/room_node_1/convective_node ==
  note: (m^3/s)
  note: (kg/s)
  note: (W)
  note: (°C)
  note: (kg water / kg air)
  note: (kg/s)
  note: (kg/s)
  note: (m^3/s)
  note: (1/s)
  note: CONVECTIVE node: absolute air mass, humidity mass, CO2 mass and air temperature in a zone
  note: (kg/m^3)
  note: SIMPLIFICATIONS:
      | 1) air in zone is incompressible
      | 2) density(dry air) = density(humid air)
      | 3) density and heat-capacity are constant
  note: (J/(kg*K))
  note: (kg CO2 / kg air)
  note: (N/m^2)
  Qdotc : Inport
  mdot_air : Inport  Port=2
  mdot_H2O : Inport  Port=3
  mdot_CO2 : Inport  Port=4
  Vdot_out2in : Inport  Port=5
  Vdot_in2out : Inport  Port=6
  (1/m^3) : Constant  Value=1/zoneairvolume
  (1/m^3)1 : Constant  Value=heatperfect
  Mean : Subsystem
  Multiport Switch : MultiPortSwitch  Inputs=2  SaturateOnIntegerOverflow=on  InputSameDT=on
  Repeating Sequence : simulink/Sources/Repeating Sequence  rep_seq_t=lookuptime  rep_seq_y=lookupvalue
  Subsystem : Subsystem
  Tair : Integrator  InitialCondition=zonestartTEMP
  Transfer Fcn (with initial outputs) : simulink_extras/Additional Linear/Transfer Fcn (with initial outputs)  N=[1]  D=[timeconst 1]  Y0=1e5  U0=0
  density_air : Constant  Value=density(zonestartTEMP, AirPressure, 2, zonestartWATER)
  heat_capacity_air : Constant  Value=heat_capacity(zonestartTEMP, AirPressure, 2, zonestartWATER)
  m_CO2 : Integrator  InitialCondition=zonestartCO2  LimitOutput=on  LowerSaturationLimit=0
  m_H2O : Integrator  InitialCondition=zonestartWATER  LimitOutput=on  LowerSaturationLimit=0
  m_air : Integrator  InitialCondition=zonestartAIR  LimitOutput=on  LowerSaturationLimit=0
  x : Product  Inputs=***  SaturateOnIntegerOverflow=on  InputSameDT=on  OutDataTypeStr=Inherit: Same as first input
  x1 : Product  Inputs=**/  SaturateOnIntegerOverflow=on  InputSameDT=on  OutDataTypeStr=Inherit: Same as first input
  x2 : Product  Inputs=**/  SaturateOnIntegerOverflow=on  InputSameDT=on  OutDataTypeStr=Inherit: Same as first input
  x3 : Product  Inputs=**//  SaturateOnIntegerOverflow=on  InputSameDT=on  OutDataTypeStr=Inherit: Same as first input
  x4 : Product  Inputs=**  SaturateOnIntegerOverflow=on  InputSameDT=on  OutDataTypeStr=Inherit: Same as first input
  Tc : Outport
  x_H2O : Outport  Port=2
  x_CO2 : Outport  Port=3
  rho : Outport  Port=4
  cp : Outport  Port=5
  p : Outport  Port=6
  nair_out : Outport  Port=7
  wires:
  Transfer Fcn (with initial outputs)/1 -> p/1
  density_air/1 -> rho/1, x3/3, x1/3, x2/3
  Qdotc/1 -> x3/1
  Mean/1(Mean) -> x4/2
  Vdot_out2in/1 -> Mean/1(u1)
  Vdot_in2out/1 -> Mean/2(u2)
  x4/1 -> nair_out/1
  x/1 -> Transfer Fcn (with initial outputs)/1
  m_H2O/1 -> x1/1
  mdot_CO2/1 -> m_CO2/1
  mdot_H2O/1 -> m_H2O/1
  x1/1 -> x_H2O/1
  Subsystem/1(R*T ') -> x/3
  mdot_air/1 -> m_air/1
  m_air/1 -> x/1
  heat_capacity_air/1 -> x3/4, cp/1
  m_CO2/1 -> x2/1
  (1/m^3)/1 -> x2/2, x/2, x1/2, x3/2, x4/1
  x3/1 -> Tair/1
  Tair/1 -> Multiport Switch/2
  x2/1 -> x_CO2/1
  Multiport Switch/1 -> Subsystem/1(T), Tc/1
  (1/m^3)1/1 -> Multiport Switch/1
  Repeating Sequence/1 -> Multiport Switch/3

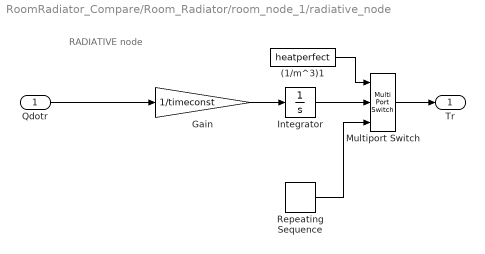
== system RoomRadiator_Compare/Room_Radiator/room_node_1/radiative_node ==
  note: RADIATIVE node
  Qdotr : Inport
  (1/m^3)1 : Constant  Value=heatperfect
  Gain : Gain  Gain=1/timeconst
  Integrator : Integrator  InitialCondition=zonestartTEMP
  Multiport Switch : MultiPortSwitch  Inputs=2  SaturateOnIntegerOverflow=on  InputSameDT=on
  Repeating Sequence : simulink/Sources/Repeating Sequence  rep_seq_t=lookuptime  rep_seq_y=lookupvalue
  Tr : Outport
  wires:
  Multiport Switch/1 -> Tr/1
  Integrator/1 -> Multiport Switch/2
  (1/m^3)1/1 -> Multiport Switch/1
  Qdotr/1 -> Gain/1
  Gain/1 -> Integrator/1
  Repeating Sequence/1 -> Multiport Switch/3

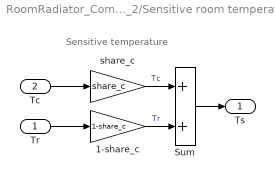
== system RoomRadiator_Compare/Room_Radiator/room_node_2/Sensitive room temperature ==
  note: Sensitive temperature
  Tr : Inport
  Tc : Inport  Port=2
  1-share_c : Gain  Gain=1-share_c  SaturateOnIntegerOverflow=on  OutDataTypeStr=Inherit: Same as input  ParamDataTypeStr=Inherit: Same as input
  Sum : Sum  SaturateOnIntegerOverflow=on  InputSameDT=on  OutDataTypeStr=Inherit: Same as first input
  share_c : Gain  Gain=share_c  SaturateOnIntegerOverflow=on  OutDataTypeStr=Inherit: Same as input  ParamDataTypeStr=Inherit: Same as input
  Ts : Outport
  wires:
  Tr/1 -> 1-share_c/1
  Tc/1 -> share_c/1
  share_c/1 -> Sum/1  "Tc"
  1-share_c/1 -> Sum/2  "Tr"
  Sum/1 -> Ts/1

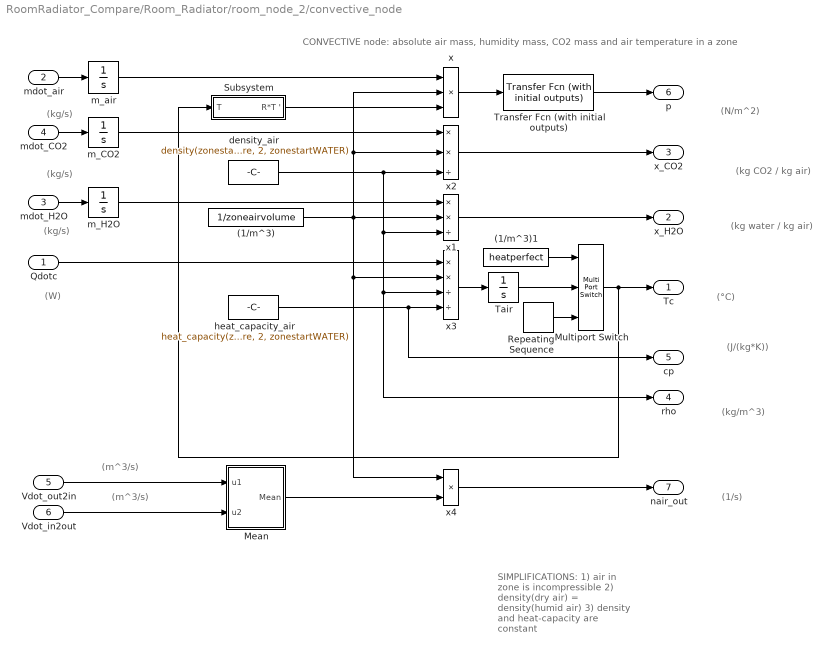
== system RoomRadiator_Compare/Room_Radiator/room_node_2/convective_node ==
  note: (m^3/s)
  note: (kg/s)
  note: (W)
  note: (°C)
  note: (kg water / kg air)
  note: (kg/s)
  note: (kg/s)
  note: (m^3/s)
  note: (1/s)
  note: CONVECTIVE node: absolute air mass, humidity mass, CO2 mass and air temperature in a zone
  note: (kg/m^3)
  note: SIMPLIFICATIONS:
      | 1) air in zone is incompressible
      | 2) density(dry air) = density(humid air)
      | 3) density and heat-capacity are constant
  note: (J/(kg*K))
  note: (kg CO2 / kg air)
  note: (N/m^2)
  Qdotc : Inport
  mdot_air : Inport  Port=2
  mdot_H2O : Inport  Port=3
  mdot_CO2 : Inport  Port=4
  Vdot_out2in : Inport  Port=5
  Vdot_in2out : Inport  Port=6
  (1/m^3) : Constant  Value=1/zoneairvolume
  (1/m^3)1 : Constant  Value=heatperfect
  Mean : Subsystem
  Multiport Switch : MultiPortSwitch  Inputs=2  SaturateOnIntegerOverflow=on  InputSameDT=on
  Repeating Sequence : simulink/Sources/Repeating Sequence  rep_seq_t=lookuptime  rep_seq_y=lookupvalue
  Subsystem : Subsystem
  Tair : Integrator  InitialCondition=zonestartTEMP
  Transfer Fcn (with initial outputs) : simulink_extras/Additional Linear/Transfer Fcn (with initial outputs)  N=[1]  D=[timeconst 1]  Y0=1e5  U0=0
  density_air : Constant  Value=density(zonestartTEMP, AirPressure, 2, zonestartWATER)
  heat_capacity_air : Constant  Value=heat_capacity(zonestartTEMP, AirPressure, 2, zonestartWATER)
  m_CO2 : Integrator  InitialCondition=zonestartCO2  LimitOutput=on  LowerSaturationLimit=0
  m_H2O : Integrator  InitialCondition=zonestartWATER  LimitOutput=on  LowerSaturationLimit=0
  m_air : Integrator  InitialCondition=zonestartAIR  LimitOutput=on  LowerSaturationLimit=0
  x : Product  Inputs=***  SaturateOnIntegerOverflow=on  InputSameDT=on  OutDataTypeStr=Inherit: Same as first input
  x1 : Product  Inputs=**/  SaturateOnIntegerOverflow=on  InputSameDT=on  OutDataTypeStr=Inherit: Same as first input
  x2 : Product  Inputs=**/  SaturateOnIntegerOverflow=on  InputSameDT=on  OutDataTypeStr=Inherit: Same as first input
  x3 : Product  Inputs=**//  SaturateOnIntegerOverflow=on  InputSameDT=on  OutDataTypeStr=Inherit: Same as first input
  x4 : Product  Inputs=**  SaturateOnIntegerOverflow=on  InputSameDT=on  OutDataTypeStr=Inherit: Same as first input
  Tc : Outport
  x_H2O : Outport  Port=2
  x_CO2 : Outport  Port=3
  rho : Outport  Port=4
  cp : Outport  Port=5
  p : Outport  Port=6
  nair_out : Outport  Port=7
  wires:
  Transfer Fcn (with initial outputs)/1 -> p/1
  density_air/1 -> rho/1, x3/3, x1/3, x2/3
  Qdotc/1 -> x3/1
  Mean/1(Mean) -> x4/2
  Vdot_out2in/1 -> Mean/1(u1)
  Vdot_in2out/1 -> Mean/2(u2)
  x4/1 -> nair_out/1
  x/1 -> Transfer Fcn (with initial outputs)/1
  m_H2O/1 -> x1/1
  mdot_CO2/1 -> m_CO2/1
  mdot_H2O/1 -> m_H2O/1
  x1/1 -> x_H2O/1
  Subsystem/1(R*T ') -> x/3
  mdot_air/1 -> m_air/1
  m_air/1 -> x/1
  heat_capacity_air/1 -> x3/4, cp/1
  m_CO2/1 -> x2/1
  (1/m^3)/1 -> x2/2, x/2, x1/2, x3/2, x4/1
  x3/1 -> Tair/1
  Tair/1 -> Multiport Switch/2
  x2/1 -> x_CO2/1
  Multiport Switch/1 -> Subsystem/1(T), Tc/1
  (1/m^3)1/1 -> Multiport Switch/1
  Repeating Sequence/1 -> Multiport Switch/3

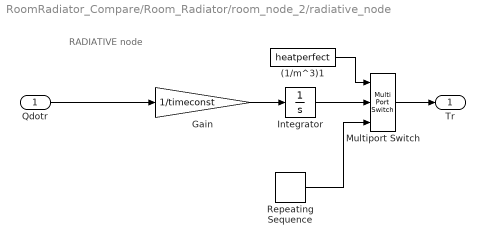
== system RoomRadiator_Compare/Room_Radiator/room_node_2/radiative_node ==
  note: RADIATIVE node
  Qdotr : Inport
  (1/m^3)1 : Constant  Value=heatperfect
  Gain : Gain  Gain=1/timeconst
  Integrator : Integrator  InitialCondition=zonestartTEMP
  Multiport Switch : MultiPortSwitch  Inputs=2  SaturateOnIntegerOverflow=on  InputSameDT=on
  Repeating Sequence : simulink/Sources/Repeating Sequence  rep_seq_t=lookuptime  rep_seq_y=lookupvalue
  Tr : Outport
  wires:
  Multiport Switch/1 -> Tr/1
  Integrator/1 -> Multiport Switch/2
  (1/m^3)1/1 -> Multiport Switch/1
  Qdotr/1 -> Gain/1
  Gain/1 -> Integrator/1
  Repeating Sequence/1 -> Multiport Switch/3

== system RoomRadiator_Compare/Room_Radiator/room_node_1/convective_node/Mean ==
  u1 : Inport
  u2 : Inport  Port=2
  Sum : Sum  SaturateOnIntegerOverflow=on  InputSameDT=on  OutDataTypeStr=Inherit: Same as first input
  gain : Gain  Gain=0.5  SaturateOnIntegerOverflow=on  OutDataTypeStr=Inherit: Same as input  ParamDataTypeStr=Inherit: Same as input
  Mean : Outport
  wires:
  u2/1 -> Sum/2
  gain/1 -> Mean/1
  u1/1 -> Sum/1
  Sum/1 -> gain/1

== system RoomRadiator_Compare/Room_Radiator/room_node_1/convective_node/Subsystem ==
  note: (J/(kg*K)
  T : Inport
  Celsius2Kelvin : Bias  Bias=273.15
  air_gas_constant : Gain  Gain=287  SaturateOnIntegerOverflow=on  OutDataTypeStr=Inherit: Same as input  ParamDataTypeStr=Inherit: Same as input
  R*T ' : Outport
  wires:
  Celsius2Kelvin/1 -> air_gas_constant/1
  T/1 -> Celsius2Kelvin/1
  air_gas_constant/1 -> R*T '/1

== system RoomRadiator_Compare/Room_Radiator/room_node_2/convective_node/Mean ==
  u1 : Inport
  u2 : Inport  Port=2
  Sum : Sum  SaturateOnIntegerOverflow=on  InputSameDT=on  OutDataTypeStr=Inherit: Same as first input
  gain : Gain  Gain=0.5  SaturateOnIntegerOverflow=on  OutDataTypeStr=Inherit: Same as input  ParamDataTypeStr=Inherit: Same as input
  Mean : Outport
  wires:
  u2/1 -> Sum/2
  gain/1 -> Mean/1
  u1/1 -> Sum/1
  Sum/1 -> gain/1

== system RoomRadiator_Compare/Room_Radiator/room_node_2/convective_node/Subsystem ==
  note: (J/(kg*K)
  T : Inport
  Celsius2Kelvin : Bias  Bias=273.15
  air_gas_constant : Gain  Gain=287  SaturateOnIntegerOverflow=on  OutDataTypeStr=Inherit: Same as input  ParamDataTypeStr=Inherit: Same as input
  R*T ' : Outport
  wires:
  Celsius2Kelvin/1 -> air_gas_constant/1
  T/1 -> Celsius2Kelvin/1
  air_gas_constant/1 -> R*T '/1
